simulink model "DSPB_MB_SS"  (Simulink 8.1)
settings: Solver=VariableStepDiscrete  StartTime=0.0  StopTime=DSPB_MB_SS_param.endTime  RelTol=1e-3
PreLoadFcn:
  | % Run the setup script when the model is opened
  | setup_DSPB_MB_SS;
InitFcn:
  | % Run the setup script again just before the
  | % model is run, so that any updates made
  | % after opening are applied.
  | setup_DSPB_MB_SS;
undefined symbols (not defined in the file or in its folder): a, AdvDSPBDMemDisplay, dpoly, DSPB_MB_SS_param, dspba, evalAionMaskParam, primtype, UseDontCare, value, x, y
libraries: DSPBAPrim x298, DspbAdvFftLibrary x34, DSPBABase x5, simulink x3, DSPBAModelBus x3, DSPBAVectorUtil x3, DSPBAControl x2
(part 1 of 4)
Description:
  | DSP Builder Advanced Template for Template Design implementing Primitive Subsystems
settings Model: Creator=mjervis  LastModifiedBy=AliReza
settings DataIOCC: SignalLoggingSaveFormat=Dataset
settings DebuggingCC: InheritedTsInSrcMsg=none  IntegerOverflowMsg=none  FcnCallInpInsideContextMsg=EnableAllAsError  FrameProcessingCompatibilityMsg=error
settings GRTTargetCC: CodeReplacementLibrary=None  CPPClassGenCompliant=on

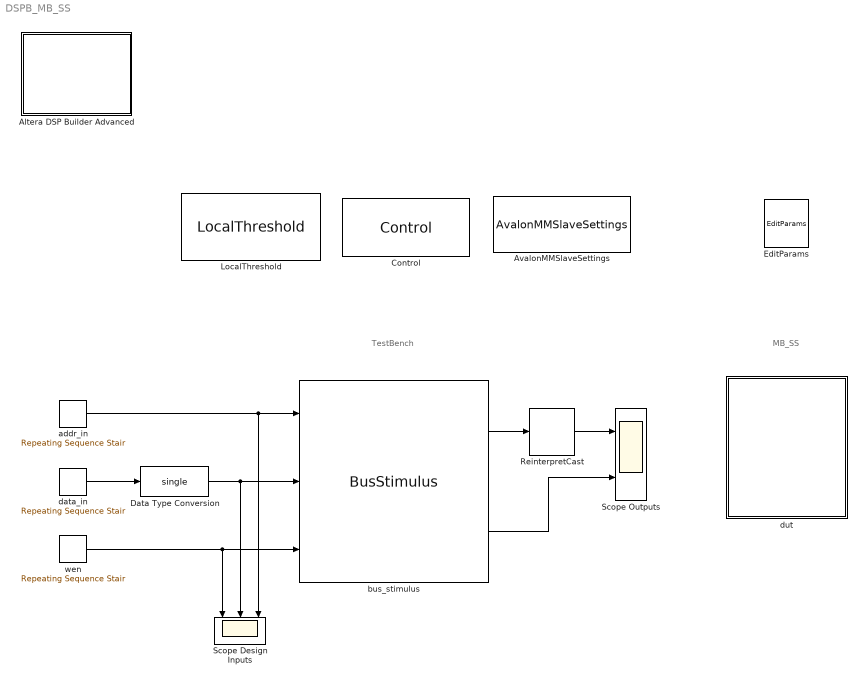
== system DSPB_MB_SS ==
  note: TestBench
  note: MB_SS
  Altera DSP Builder Advanced : Subsystem  mask(DSP Builder Advanced Blockset Ignored Block){}
      settings: OpenFcn=web('http://www.altera.com', '-new');
      mask Display: image(imread('intellogo.tif'));
  AvalonMMSlaveSettings : DSPBABase/AvalonMMSlaveSettings
  "Control " : DSPBABase/Control  generate=on  language=VHDL  destination=./rtl  make_full_path=off  path_is_relative=on  autotestbench=on  signaldepth=2  coveragetestbench=off  logs=off  spacewidth=2  spacenum=1  addrwidth=10  datawidth=16  dataendian=Big Endian  hierarchicalnames=on  ramThresholdBits=-1  distRamThresholdBits=-1  mlabThresholdBits=-1  hardMultiplierThresholdLuts=-1  version=20090407  errorOnChanMismatch=1  errorOnGPIOMismatch=0  importModelsimResults=0  cycleAccurate=off  reinterpretCastMult=off  paramFile=DSPB_MB_SS_params.xml
  Data Type Conversion : DataTypeConversion  OutDataTypeStr=single
  EditParams : DSPBABase/EditParams  version=20090407
  LocalThreshold : DSPBABase/LocalThreshold  margin=0  delayRegOrRAMThresholdBits=-1  MediumDualMemThresholdBits=-1  LargeDualMemThresholdBits=0  hardMultiplierThresholdLuts=0  complexMultKaratsuba=off  version=0
  ReinterpretCast : DSPBAPrim/ReinterpretCast  primtype=reinterpret  nInputs=1  nOutputs=1  omode=single  otype=sfix(16)  scale=2^-15  rndmethod=Unbiased  factor=1  satmethod=Symmetric  shift_vec=[0 1 2 -1]  value=0  inPortNames=[' '; ' ';]  outPortNames=[' ']  dspbaimage=dspba_prim.jpg  text=fprintf('Reinterp\nCast', value);  style=Optimised  visibilities=8  floatPrecision=float32_m23  version=20120601
  Scope Outputs : Scope  NumInputPorts=2
  Scope Design Inputs : Scope  NumInputPorts=3
  addr_in : simulink/Sources/Repeating Sequence Stair  OutValues=DSPB_MB_SS_IO.bus_addr_in  tsamp=1  OutMin=[]  OutMax=[]  OutDataTypeStr=Inherit: Inherit via back propagation  OutDataType=fixdt(0,3)  ConRadixGroup=Best Precision: Vector-wise  OutScaling=[]
  bus_stimulus : DSPBAModelBus/BusStimulus  SampleTime=-1  version=20140122  hasreaden=off
  data_in : simulink/Sources/Repeating Sequence Stair  OutValues=DSPB_MB_SS_IO.bus_data_in  tsamp=1  OutMin=[]  OutMax=[]  OutDataTypeStr=double  OutputDataTypeScalingMode=double  OutDataType=fixdt(0,3)  ConRadixGroup=Best Precision: Vector-wise  OutScaling=[]
  dut : Subsystem
  wen : simulink/Sources/Repeating Sequence Stair  OutValues=DSPB_MB_SS_IO.bus_wen  tsamp=1  OutMin=[]  OutMax=[]  OutDataTypeStr=fixdt('boolean')  OutputDataTypeScalingMode=Specify via dialog  OutDataType=fixdt('boolean')  ConRadixGroup=Best Precision: Vector-wise  OutScaling=[]
  wires:
  bus_stimulus/2 -> Scope Outputs/2
  addr_in/1 -> Scope Design Inputs/3, bus_stimulus/1
  wen/1 -> Scope Design Inputs/1, bus_stimulus/3
  data_in/1 -> Data Type Conversion/1
  Data Type Conversion/1 -> Scope Design Inputs/2, bus_stimulus/2
  bus_stimulus/1 -> ReinterpretCast/1
  ReinterpretCast/1 -> Scope Outputs/1

== system DSPB_MB_SS/Altera DSP Builder Advanced ==

== system DSPB_MB_SS/dut ==
  Device : DSPBABase/Device  family=Arria 10  stratix4device=Stratix IV E  hardcopy4device=HardCopy IV E  stratix5device=Stratix V GX  device=AUTO  speed=1  stratixSpeed=-5  stratix2Speed=-3  stratix3Speed=-2  stratix4gxSpeed=-2  stratix4gtSpeed=-1  cyclone2Speed=-6  cyclone3Speed=-7  arria2Speed=-4  cyclone4eSpeed=-8  stratix5Speed=-3  arria5Speed=-4  arriaSpeed=-6  cyclone3lsSpeed=-7  cyclone5Speed=-6  arria2gzSpeed=-3  nightFurySpeed=-2  ecp2Speed=-7  hardcopycompat=off  version=20140217  max10flashmode=off  max10nomeminit=off
  Enhacement_Algorithm_MB_SS : Subsystem
  Feature_Extraction : Subsystem
  Input_Interface : Subsystem
  Output_Interface : Subsystem
  wires:
  Feature_Extraction/1(Noisy_Signal_Power_Spectrum_Valid) -> Enhacement_Algorithm_MB_SS/1(Signal_Power_Spectrum_valid)
  Feature_Extraction/2(Noisy_Signal_Power_Spectrum) -> Enhacement_Algorithm_MB_SS/2(Signal_Power_Spectrum)
  Feature_Extraction/3(Noise_Power_Spectrum_Valid) -> Enhacement_Algorithm_MB_SS/3(Noise_Power_Spectrum_Valid)
  Feature_Extraction/5(Noisy_Signal_Phase_Valid) -> Enhacement_Algorithm_MB_SS/5(Signal_Phase_Valid)
  Feature_Extraction/6(Noisy_Signal_Phase) -> Enhacement_Algorithm_MB_SS/6(Signal_Phase)
  Enhacement_Algorithm_MB_SS/1(Enhanced_Signal_Valid) -> Output_Interface/1(Enhanced_Signal_Valid)
  Enhacement_Algorithm_MB_SS/2(Enhanced_Signal) -> Output_Interface/2(Enhanced_Signal)
  Input_Interface/1(Noisy_Signal_Valid) -> Feature_Extraction/1(Input_Signal_Valid)
  Feature_Extraction/4(Noise_Power_Spectrum) -> Enhacement_Algorithm_MB_SS/4(Noise_Power_Spectrum)
  Input_Interface/2(Noisy_Signal) -> Feature_Extraction/2(Input_Signal)

== system DSPB_MB_SS/dut/Enhacement_Algorithm_MB_SS ==
  Signal_Power_Spectrum_valid : Inport
  Signal_Power_Spectrum : Inport  Port=2
  Noise_Power_Spectrum_Valid : Inport  Port=3
  Noise_Power_Spectrum : Inport  Port=4
  Signal_Phase_Valid : Inport  Port=5
  Signal_Phase : Inport  Port=6
  MultiBand_Spectral_Subtraction : Subsystem
  Time_Domain_Reconstruction : Subsystem
  Enhanced_Signal_Valid : Outport
  Enhanced_Signal : Outport  Port=2
  wires:
  Time_Domain_Reconstruction/1(Time_Domain_Output_Valid) -> Enhanced_Signal_Valid/1
  Time_Domain_Reconstruction/2(Time_Domain_Output) -> Enhanced_Signal/1
  MultiBand_Spectral_Subtraction/1(Enhanced_Magnitude_Spectrum) -> Time_Domain_Reconstruction/1(Enhanced_Magnitude_Spectrum)
  MultiBand_Spectral_Subtraction/2(Enhanced_Magnitude_Spectrum_Valid) -> Time_Domain_Reconstruction/2(Enhanced_Magnitude_Spectrum_Valid)
  Noise_Power_Spectrum/1 -> MultiBand_Spectral_Subtraction/4(Noise_Power)
  Noise_Power_Spectrum_Valid/1 -> MultiBand_Spectral_Subtraction/3(Noise_Power_Valid)
  Signal_Power_Spectrum/1 -> MultiBand_Spectral_Subtraction/2(Signal_Power)
  Signal_Power_Spectrum_valid/1 -> MultiBand_Spectral_Subtraction/1(Signal_Power_Valid)
  Signal_Phase_Valid/1 -> Time_Domain_Reconstruction/3(Phase_Valid)
  Signal_Phase/1 -> Time_Domain_Reconstruction/4(Phase)

== system DSPB_MB_SS/dut/Feature_Extraction ==
  Input_Signal_Valid : Inport
  Input_Signal : Inport  Port=2
  A_Posteriori_SNR : Subsystem
  FFT : Subsystem
  FFT_Adapter : Subsystem
  Noisy_Signal_Power_Spectrum_Valid : Outport
  Noisy_Signal_Power_Spectrum : Outport  Port=2
  Noise_Power_Spectrum_Valid : Outport  Port=3
  Noise_Power_Spectrum : Outport  Port=4
  Noisy_Signal_Phase_Valid : Outport  Port=5
  Noisy_Signal_Phase : Outport  Port=6
  wires:
  FFT/1(_Valid) -> FFT_Adapter/1(FFT_In_Valid)
  FFT/2(Output) -> FFT_Adapter/2(FFT_In)
  A_Posteriori_SNR/1(Noise_Power_Spectrum_Valid) -> Noise_Power_Spectrum_Valid/1
  FFT_Adapter/1(Magnitude_Spectrum_Valid) -> A_Posteriori_SNR/1(Magnitude_Spectrum_Valid)
  FFT_Adapter/2(Magnitude_Spectrum) -> A_Posteriori_SNR/2(Magnitude_Spectrum)
  FFT_Adapter/5(Phase_Valid) -> Noisy_Signal_Phase_Valid/1
  FFT_Adapter/6(Phase) -> Noisy_Signal_Phase/1
  Input_Signal_Valid/1 -> FFT/1(Valid)
  Input_Signal/1 -> FFT/2(Input)
  FFT_Adapter/4(Power_Spectrum) -> Noisy_Signal_Power_Spectrum/1
  FFT_Adapter/3(Power_Spectrum_Valid) -> Noisy_Signal_Power_Spectrum_Valid/1
  A_Posteriori_SNR/2(Noise_Power_Spectrum) -> Noise_Power_Spectrum/1

== system DSPB_MB_SS/dut/Input_Interface ==
  And : DSPBAPrim/And  primtype=and  nInputs=3  nOutputs=1  omode=Inherit via internal rule  otype=sfix(16)  scale=2^-15  rndmethod=Unbiased  factor=1  satmethod=Symmetric  shift_vec=[0 1 2 -1]  value=0  inPortNames=[' '; ' '; ' '; ' '; ' '; ' '; ' '; ' '; ' '; ' '; ' '; ' '; ' '; ' '; ' '; ' '; ]  outPortNames=[' ']  dspbaimage=dspba_prim.jpg  text=fprintf('&');  style=Optimised  visibilities=8+2  version=20090407
  Const1 : DSPBAPrim/Const  primtype=const  nInputs=0  nOutputs=1  omode=Specify via dialog  otype=ufix(DSPB_MB_SS_param.FS+1)  scale=2^-0  rndmethod=Unbiased  factor=1  satmethod=Symmetric  shift_vec=[0 1 2 -1]  value=0  inPortNames=['+'; '+';]  outPortNames=[' ']  dspbaimage=dspba_prim.jpg  text=fprintf('%s', num2str(value));  style=Optimised  visibilities=8 + 1024  floatPrecision=float32_m23  version=20120820
  Const2 : DSPBAPrim/Const  primtype=const  nInputs=0  nOutputs=1  omode=single  otype=ufix(DSPB_MB_SS_param.FS+1)  scale=2^-0  rndmethod=Unbiased  factor=1  satmethod=Symmetric  shift_vec=[0 1 2 -1]  value=0  inPortNames=['+'; '+';]  outPortNames=[' ']  dspbaimage=dspba_prim.jpg  text=fprintf('%s', num2str(value));  style=Optimised  visibilities=8 + 1024  floatPrecision=float32_m23  version=20120820
  Const3 : DSPBAPrim/Const  primtype=const  nInputs=0  nOutputs=1  omode=single  otype=sfix(16)  scale=2^-15  rndmethod=Unbiased  factor=1  satmethod=Symmetric  shift_vec=[0 1 2 -1]  value=1  inPortNames=['+'; '+';]  outPortNames=[' ']  dspbaimage=dspba_prim.jpg  text=fprintf('%s', num2str(value));  style=Optimised  visibilities=8 + 1024  floatPrecision=float32_m23  version=20120820
  EdgeDetect : DspbAdvFftLibrary/Common/EdgeDetect
  GPOut : DSPBAPrim/GPOut  primtype=gpout  nInputs=evalAionMaskParam(gcb,'value',1)  nOutputs=evalAionMaskParam(gcb,'value',1)  omode=Inherit via internal rule  otype=sfix(16)  scale=2^-15  rndmethod=Unbiased  factor=1  satmethod=Symmetric  shift_vec=[0 1 2 -1]  value=2  inPortNames=[' ' ' ' ' ' ' ' ' ' ' ' ' ' ' ' ' ' ' ' ' ' ' ' ' ' ' ' ' ' ' ' ' ' ' ' ' ' ' ' ' ' ' ' ' ' ' ' ' ' ' ' ' ' ' ' ' ' ' ' ' ' ' ' ' ' ' ' ' ']'  outPortNames=[' ' ' ' ' ' ' ' ' ' ' ' ' ' ' ' ' ' ' ' ' ' ' ' ' ' ' ' ' ' ' ' ' ' ' ' ' ' ' ' ' ' ' ' ' ' ' ' ' ' ' ' ' ' ' ' ' ' ' ' ' ' ' ' ' ' ' ' ' ']'  dspbaimage=dspba_prim.jpg  text=fprintf('GPOut');  style=Optimised  visibilities=1024  latencyCorrection=0  version=20090407
  PulseMultiplier : DspbAdvFftLibrary/Common/PulseMultiplier  N=DSPB_MB_SS_param.FS
  SampleDelay : DSPBAPrim/SampleDelay  primtype=sampdelay  nInputs=1  nOutputs=1  omode=Inherit via internal rule  otype=sfix(16)  scale=2^-15  rndmethod=Unbiased  factor=1  satmethod=Symmetric  shift_vec=[0 1 2 -1]  value=3  inPortNames=[' '; ' ';]  outPortNames=[' ']  dspbaimage=dspba_prim.jpg  text=dpoly(1, eye(1,value+1), 'z')  style=Optimised  visibilities=8 + 1024 + 2^17 + 2^18  flexible=off  slackgroup=0  augmented=0  version=20090407  advOptions=[]
  SampleDelay1 : DSPBAPrim/SampleDelay  primtype=sampdelay  nInputs=1  nOutputs=1  omode=Inherit via internal rule  otype=sfix(16)  scale=2^-15  rndmethod=Unbiased  factor=1  satmethod=Symmetric  shift_vec=[0 1 2 -1]  value=1  inPortNames=[' '; ' ';]  outPortNames=[' ']  dspbaimage=dspba_prim.jpg  text=dpoly(1, eye(1,value+1), 'z')  style=Optimised  visibilities=8 + 1024 + 2^17 + 2^18  flexible=off  slackgroup=0  augmented=0  version=20090407  advOptions=[]
  SynthesisInfo : DSPBAPrim/SynthesisInfo  primtype=synthinfo  nInputs=0  nOutputs=0  omode=Inherit via internal rule  otype=sfix(16)  scale=2^-15  rndmethod=Truncate  factor=1  satmethod=Symmetric  shift_vec=[0 1 2 -1]  value=99  inPortNames=[' '; ' ';]  outPortNames=[' ']  dspbaimage=dspba_prim_ctrl.jpg  text=fprintf('Style=%s', style);  style=Scheduled  visibilities=2^17+2^18+2^19+2^20  constraintInUse=off  constraintRelation=>  constraintLimit=2  bitAccurate=off  version=20150220
  addr_counter : Subsystem
  frame_ready : DSPBAPrim/CmpEQ  primtype=cmpeq  nInputs=2  nOutputs=1  omode=boolean  otype=sfix(16)  scale=2^-15  rndmethod=Unbiased  factor=1  satmethod=Symmetric  shift_vec=[0 1 2 -1]  value=0  inPortNames=[' '; ' ';]  outPortNames=[' ']  dspbaimage=dspba_prim.jpg  text=fprintf('==');  style=Optimised  visibilities=0  advOptions=[]  version=20130117
  frame_ready1 : DSPBAPrim/CmpEQ  primtype=cmpeq  nInputs=2  nOutputs=1  omode=boolean  otype=sfix(16)  scale=2^-15  rndmethod=Unbiased  factor=1  satmethod=Symmetric  shift_vec=[0 1 2 -1]  value=0  inPortNames=[' '; ' ';]  outPortNames=[' ']  dspbaimage=dspba_prim.jpg  text=fprintf('==');  style=Optimised  visibilities=0  advOptions=[]  version=20130117
  input_fifo : DSPBAModelBus/SharedMem  mem_addr=0  mem_rwmode=Read/Write  mem_data=zeros(1,2^(DSPB_MB_SS_param.FS)+1)  mem_init=on  mem_desc=input fifo  mem_mode=single  mem_type=sfix(16)  mem_scale=2^-8  SampleTime=-1  version=20090407
  Noisy_Signal_Valid : Outport
  Noisy_Signal : Outport  Port=2
  wires:
  Const3/1 -> frame_ready/2
  And/1 -> SampleDelay/1
  SampleDelay/1 -> SampleDelay1/1, input_fifo/3
  addr_counter/1(count) -> input_fifo/1, frame_ready1/1
  SampleDelay1/1 -> PulseMultiplier/1
  frame_ready/1 -> EdgeDetect/1, And/1
  frame_ready1/1 -> And/2
  Const1/1 -> frame_ready1/2
  PulseMultiplier/1 -> GPOut/1, addr_counter/1(en)
  GPOut/2 -> Noisy_Signal/1
  EdgeDetect/1 -> And/3
  input_fifo/1 -> GPOut/2, frame_ready/1
  GPOut/1 -> Noisy_Signal_Valid/1
  Const2/1 -> input_fifo/2

== system DSPB_MB_SS/dut/Output_Interface ==
  Enhanced_Signal_Valid : Inport
  Enhanced_Signal : Inport  Port=2
  And2 : DSPBAPrim/And  primtype=and  nInputs=2  nOutputs=1  omode=Inherit via internal rule  otype=sfix(16)  scale=2^-15  rndmethod=Unbiased  factor=1  satmethod=Symmetric  shift_vec=[0 1 2 -1]  value=0  inPortNames=[' '; ' '; ' '; ' '; ' '; ' '; ' '; ' '; ' '; ' '; ' '; ' '; ' '; ' '; ' '; ' '; ]  outPortNames=[' ']  dspbaimage=dspba_prim.jpg  text=fprintf('&');  style=Optimised  visibilities=8+2  version=20090407
  Const : DSPBAPrim/Const  primtype=const  nInputs=0  nOutputs=1  omode=single  otype=sfix(16)  scale=2^-15  rndmethod=Unbiased  factor=1  satmethod=Symmetric  shift_vec=[0 1 2 -1]  value=1  inPortNames=['+'; '+';]  outPortNames=[' ']  dspbaimage=dspba_prim.jpg  text=fprintf('%s', num2str(value));  style=Optimised  visibilities=8 + 1024  floatPrecision=float32_m23  version=20120820
  DEBUG_MONITR : Subsystem  Commented=on
  EdgeDetect1 : DspbAdvFftLibrary/Common/EdgeDetect
  GPIn : DSPBAPrim/GPIn  primtype=gpin  nInputs=evalAionMaskParam(gcb,'value',1)  nOutputs=evalAionMaskParam(gcb,'value',1)  omode=Inherit via internal rule  otype=sfix(16)  scale=2^-15  rndmethod=Unbiased  factor=1  satmethod=Symmetric  shift_vec=[0 1 2 -1]  value=2  inPortNames=[' ' ' ' ' ' ' ' ' ' ' ' ' ' ' ' ' ' ' ' ' ' ' ' ' ' ' ' ' ' ' ' ' ' ' ' ' ' ' ' ' ' ' ' ' ' ' ' ' ' ' ' ' ' ' ' ' ' ' ' ' ' ' ' ' ' ' ' ' ']'  outPortNames=[' ' ' ' ' ' ' ' ' ' ' ' ' ' ' ' ' ' ' ' ' ' ' ' ' ' ' ' ' ' ' ' ' ' ' ' ' ' ' ' ' ' ' ' ' ' ' ' ' ' ' ' ' ' ' ' ' ' ' ' ' ' ' ' ' ' ' ' ' ']'  dspbaimage=dspba_prim.jpg  text=fprintf('GPIn');  style=Optimised  visibilities=1024  latencyCorrection=0  scheduleOrigin=on  version=20090407
  Mux : DSPBAPrim/Mux  primtype=mux  nInputs=evalAionMaskParam(gcb,'value',1)+1  nOutputs=1  omode=Inherit via internal rule  otype=sfix(16)  scale=2^-15  rndmethod=Unbiased  factor=1  satmethod=Symmetric  shift_vec=[0 1 2 -1]  value=2  inPortNames=['s '; 'd0'; 'd1'; 'd2'; 'd3'; 'd4'; 'd5'; 'd6'; 'd7'; 'd8'; 'd9';]  outPortNames=[' ']  dspbaimage=dspba_prim.jpg  text=fprintf('%s', primtype);  style=Optimised  visibilities=1032  version=20131025
  Not1 : DSPBAPrim/Not  primtype=not  nInputs=1  nOutputs=1  omode=Inherit via internal rule  otype=sfix(16)  scale=2^-15  rndmethod=Unbiased  factor=1  satmethod=Symmetric  shift_vec=[0 1 2 -1]  value=0  inPortNames=[' '; ' ';]  outPortNames=[' ']  dspbaimage=dspba_prim.jpg  text=fprintf('~');  style=Optimised  visibilities=8  version=20090407
  Or : DSPBAPrim/Or  primtype=or  nInputs=2  nOutputs=1  omode=Inherit via internal rule  otype=sfix(16)  scale=2^-15  rndmethod=Unbiased  factor=1  satmethod=Symmetric  shift_vec=[0 1 2 -1]  value=0  inPortNames=[' '; ' '; ' '; ' '; ' '; ' '; ' '; ' '; ' '; ' '; ' '; ' '; ' '; ' '; ' '; ' '; ]  outPortNames=[' ']  dspbaimage=dspba_prim.jpg  text=fprintf('|');  style=Optimised  visibilities=8+2  version=20090407
  SynthesisInfo : DSPBAPrim/SynthesisInfo  primtype=synthinfo  nInputs=0  nOutputs=0  omode=Inherit via internal rule  otype=sfix(16)  scale=2^-15  rndmethod=Truncate  factor=1  satmethod=Symmetric  shift_vec=[0 1 2 -1]  value=99  inPortNames=[' '; ' ';]  outPortNames=[' ']  dspbaimage=dspba_prim_ctrl.jpg  text=fprintf('Style=%s', style);  style=Scheduled  visibilities=2^17+2^18+2^19+2^20  constraintInUse=off  constraintRelation=>  constraintLimit=2  bitAccurate=off  version=20150220
  Terminator1 : Terminator
  addr_counter1 : Subsystem
  output_fifo : DSPBAModelBus/SharedMem  mem_addr=2^(DSPB_MB_SS_param.FS)+1  mem_rwmode=Read/Write  mem_data=zeros(1,2^(DSPB_MB_SS_param.FS)+1)  mem_init=on  mem_desc=output fifo  mem_mode=single  mem_type=sfix(16)  mem_scale=2^-8  SampleTime=-1  version=20090407
  wires:
  Enhanced_Signal/1 -> GPIn/2
  Enhanced_Signal_Valid/1 -> GPIn/1
  And2/1 -> Or/1, Mux/1
  GPIn/1 -> Or/2, Not1/1, EdgeDetect1/1, addr_counter1/1(en)
  output_fifo/1 -> Terminator1/1
  EdgeDetect1/1 -> And2/1
  Const/1 -> Mux/3
  Or/1 -> DEBUG_MONITR/3(we), output_fifo/3
  Not1/1 -> And2/2
  Mux/1 -> DEBUG_MONITR/2(wd), output_fifo/2
  GPIn/2 -> Mux/2
  addr_counter1/1(count) -> output_fifo/1, DEBUG_MONITR/1(addr)

== system DSPB_MB_SS/dut/Enhacement_Algorithm_MB_SS/MultiBand_Spectral_Subtraction ==
  note: S. D. Kamath and P. C. Loizou, “A MULTI-BAND SPECTRAL SUBTRACTION METHOD FOR ENHANCING SPEECH CORRUPTED BY COLORED NOISE,” p. 4.
  Signal_Power_Valid : Inport
  Signal_Power : Inport  Port=2
  Noise_Power_Valid : Inport  Port=3
  Noise_Power : Inport  Port=4
  Alpha : Subsystem
  MB_SS_Core : Subsystem
  Enhanced_Magnitude_Spectrum : Outport
  Enhanced_Magnitude_Spectrum_Valid : Outport  Port=2
  wires:
  Signal_Power/1 -> MB_SS_Core/2(Signal_Power), Alpha/2(Signal_Power)
  Signal_Power_Valid/1 -> MB_SS_Core/1(Signal_Power_Valid), Alpha/1(Signal_Power_Valid)
  Noise_Power_Valid/1 -> MB_SS_Core/3(Noise_Power_Valid), Alpha/3(Noise_Power_Valid)
  Noise_Power/1 -> MB_SS_Core/4(Noise_Power), Alpha/4(Noise_Power)
  Alpha/1(Valid) -> MB_SS_Core/5(Alpha_Valid)
  MB_SS_Core/1(Enhanced_Magnitude_Valid) -> Enhanced_Magnitude_Spectrum_Valid/1
  MB_SS_Core/2(Enhanced_Magnitude) -> Enhanced_Magnitude_Spectrum/1
  Alpha/2(Alpha) -> MB_SS_Core/6(Alpha)

== system DSPB_MB_SS/dut/Enhacement_Algorithm_MB_SS/Time_Domain_Reconstruction ==
  Enhanced_Magnitude_Spectrum : Inport
  Enhanced_Magnitude_Spectrum_Valid : Inport  Port=2
  Phase_Valid : Inport  Port=3
  Phase : Inport  Port=4
  IFFT : Subsystem
  IFFT_Adapter : Subsystem
  Time_Domain_Output_Valid : Outport
  Time_Domain_Output : Outport  Port=2
  wires:
  IFFT/2(Time_Domain_Output) -> Time_Domain_Output/1
  Enhanced_Magnitude_Spectrum_Valid/1 -> IFFT_Adapter/2(Enhanced_Magnitude_Valid)
  IFFT/1(Time_Domain_Output_Valid) -> Time_Domain_Output_Valid/1
  IFFT_Adapter/1(Output_Valid) -> IFFT/1(Input_Valid)
  IFFT_Adapter/2(Output) -> IFFT/2(Input)
  Enhanced_Magnitude_Spectrum/1 -> IFFT_Adapter/3(Enhanced_Magnitude)
  Phase_Valid/1 -> IFFT_Adapter/1(Phase_Valid)
  Phase/1 -> IFFT_Adapter/4(Phase)

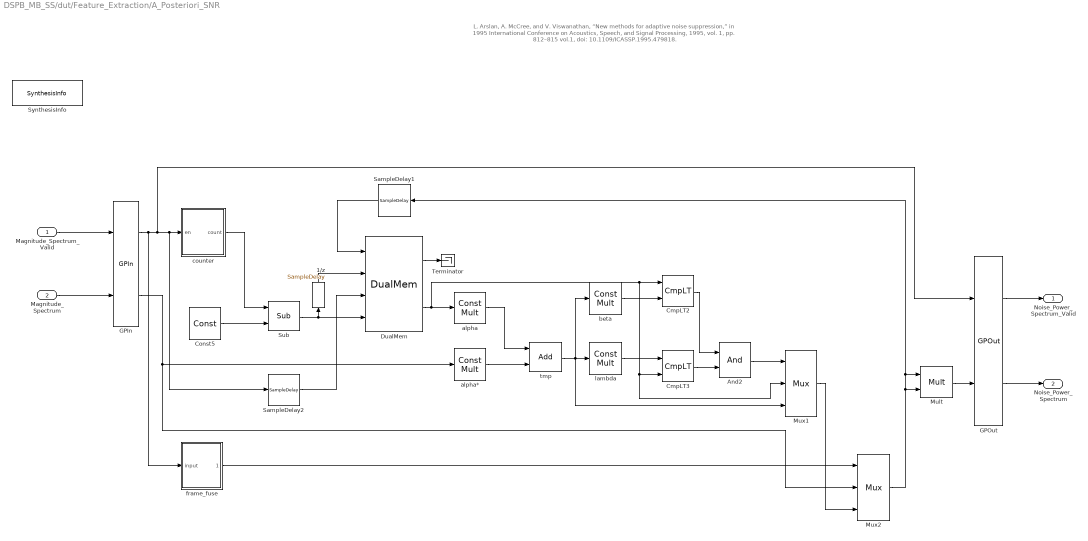
== system DSPB_MB_SS/dut/Feature_Extraction/A_Posteriori_SNR ==
  note: L. Arslan, A. McCree, and V. Viswanathan, “New methods for adaptive noise suppression,”
      |  in 1995 International Conference on Acoustics, Speech, and Signal Processing, 1995,
      | vol. 1, pp. 812–815 vol.1, doi: 10.1109/ICASSP.1995.479818.
  Magnitude_Spectrum_Valid : Inport
  Magnitude_Spectrum : Inport  Port=2
  1/z : DSPBAPrim/SampleDelay  primtype=sampdelay  nInputs=1  nOutputs=1  omode=Inherit via internal rule  otype=sfix(16)  scale=2^-15  rndmethod=Unbiased  factor=1  satmethod=Symmetric  shift_vec=[0 1 2 -1]  value=6  inPortNames=[' '; ' ';]  outPortNames=[' ']  dspbaimage=dspba_prim.jpg  text=dpoly(1, eye(1,value+1), 'z')  style=Optimised  visibilities=8 + 1024 + 2^17 + 2^18  flexible=off  slackgroup=0  augmented=0  version=20090407  advOptions=[]
  And2 : DSPBAPrim/And  primtype=and  nInputs=2  nOutputs=1  omode=Inherit via internal rule  otype=sfix(16)  scale=2^-15  rndmethod=Unbiased  factor=1  satmethod=Symmetric  shift_vec=[0 1 2 -1]  value=0  inPortNames=[' '; ' '; ' '; ' '; ' '; ' '; ' '; ' '; ' '; ' '; ' '; ' '; ' '; ' '; ' '; ' '; ]  outPortNames=[' ']  dspbaimage=dspba_prim.jpg  text=fprintf('&');  style=Optimised  visibilities=8+2  version=20090407
  CmpLT2 : DSPBAPrim/CmpLT  primtype=cmplt  nInputs=2  nOutputs=1  omode=boolean  otype=sfix(16)  scale=2^-15  rndmethod=Unbiased  factor=1  satmethod=Symmetric  shift_vec=[0 1 2 -1]  value=0  inPortNames=['a'; 'b';]  outPortNames=[' ']  dspbaimage=dspba_prim.jpg  text=fprintf('a<b');  style=Optimised  visibilities=0  advOptions=[]  version=20130117
  CmpLT3 : DSPBAPrim/CmpLT  primtype=cmplt  nInputs=2  nOutputs=1  omode=boolean  otype=sfix(16)  scale=2^-15  rndmethod=Unbiased  factor=1  satmethod=Symmetric  shift_vec=[0 1 2 -1]  value=0  inPortNames=['a'; 'b';]  outPortNames=[' ']  dspbaimage=dspba_prim.jpg  text=fprintf('a<b');  style=Optimised  visibilities=0  advOptions=[]  version=20130117
  Const5 : DSPBAPrim/Const  primtype=const  nInputs=0  nOutputs=1  omode=Specify via dialog  otype=ufix(DSPB_MB_SS_param.FS+1)  scale=2^-0  rndmethod=Unbiased  factor=1  satmethod=Symmetric  shift_vec=[0 1 2 -1]  value=1  inPortNames=['+'; '+';]  outPortNames=[' ']  dspbaimage=dspba_prim.jpg  text=fprintf('%s', num2str(value));  style=Optimised  visibilities=8 + 1024  floatPrecision=float32_m23  version=20120820
  DualMem : DSPBAPrim/DualMem  primtype=dualmem  nInputs=4  nOutputs=2  omode=single  otype=sfix(16)  scale=2^-15  rndmethod=Unbiased  factor=1  satmethod=Symmetric  shift_vec=[0 1 2 -1]  value=[zeros(2^DSPB_MB_SS_param.FS, 1)]  inPortNames=['d1'; 'a1'; 'w1'; 'a2']  outPortNames=['q1'; 'q2']  dspbaimage=dspba_prim.jpg  text=fprintf('dmem%s',AdvDSPBDMemDisplay(UseDontCare));  style=Optimised  visibilities=8 + 1024 + 2^17 + 2^18  UseDontCare=on  TwinWritePorts=off  version=20141001
  GPIn : DSPBAPrim/GPIn  primtype=gpin  nInputs=evalAionMaskParam(gcb,'value',1)  nOutputs=evalAionMaskParam(gcb,'value',1)  omode=Inherit via internal rule  otype=sfix(16)  scale=2^-15  rndmethod=Unbiased  factor=1  satmethod=Symmetric  shift_vec=[0 1 2 -1]  value=2  inPortNames=[' ' ' ' ' ' ' ' ' ' ' ' ' ' ' ' ' ' ' ' ' ' ' ' ' ' ' ' ' ' ' ' ' ' ' ' ' ' ' ' ' ' ' ' ' ' ' ' ' ' ' ' ' ' ' ' ' ' ' ' ' ' ' ' ' ' ' ' ' ']'  outPortNames=[' ' ' ' ' ' ' ' ' ' ' ' ' ' ' ' ' ' ' ' ' ' ' ' ' ' ' ' ' ' ' ' ' ' ' ' ' ' ' ' ' ' ' ' ' ' ' ' ' ' ' ' ' ' ' ' ' ' ' ' ' ' ' ' ' ' ' ' ' ']'  dspbaimage=dspba_prim.jpg  text=fprintf('GPIn');  style=Optimised  visibilities=1024  latencyCorrection=0  scheduleOrigin=on  version=20090407
  GPOut : DSPBAPrim/GPOut  primtype=gpout  nInputs=evalAionMaskParam(gcb,'value',1)  nOutputs=evalAionMaskParam(gcb,'value',1)  omode=Inherit via internal rule  otype=sfix(16)  scale=2^-15  rndmethod=Unbiased  factor=1  satmethod=Symmetric  shift_vec=[0 1 2 -1]  value=2  inPortNames=[' ' ' ' ' ' ' ' ' ' ' ' ' ' ' ' ' ' ' ' ' ' ' ' ' ' ' ' ' ' ' ' ' ' ' ' ' ' ' ' ' ' ' ' ' ' ' ' ' ' ' ' ' ' ' ' ' ' ' ' ' ' ' ' ' ' ' ' ' ']'  outPortNames=[' ' ' ' ' ' ' ' ' ' ' ' ' ' ' ' ' ' ' ' ' ' ' ' ' ' ' ' ' ' ' ' ' ' ' ' ' ' ' ' ' ' ' ' ' ' ' ' ' ' ' ' ' ' ' ' ' ' ' ' ' ' ' ' ' ' ' ' ' ']'  dspbaimage=dspba_prim.jpg  text=fprintf('GPOut');  style=Optimised  visibilities=1024  latencyCorrection=0  version=20090407
  Mult : DSPBAPrim/Mult  primtype=mult  nInputs=2  nOutputs=1  omode=Inherit via internal rule  otype=sfix(16)  scale=2^-15  rndmethod=Unbiased  factor=1  satmethod=Symmetric  shift_vec=[0 1 2 -1]  value=0  inPortNames=[' '; ' ';]  outPortNames=[' ']  dspbaimage=dspba_prim.jpg  text=fprintf('X');  style=Optimised  visibilities=8+2^18+2^19  floatPrecision=float32_m23  floatRounding=correct  advOptions=[]  version=20130115
  Mux1 : DSPBAPrim/Mux  primtype=mux  nInputs=evalAionMaskParam(gcb,'value',1)+1  nOutputs=1  omode=Inherit via internal rule  otype=sfix(16)  scale=2^-15  rndmethod=Unbiased  factor=1  satmethod=Symmetric  shift_vec=[0 1 2 -1]  value=2  inPortNames=['s '; 'd0'; 'd1'; 'd2'; 'd3'; 'd4'; 'd5'; 'd6'; 'd7'; 'd8'; 'd9';]  outPortNames=[' ']  dspbaimage=dspba_prim.jpg  text=fprintf('%s', primtype);  style=Optimised  visibilities=1032  version=20131025
  Mux2 : DSPBAPrim/Mux  primtype=mux  nInputs=evalAionMaskParam(gcb,'value',1)+1  nOutputs=1  omode=Inherit via internal rule  otype=sfix(16)  scale=2^-15  rndmethod=Unbiased  factor=1  satmethod=Symmetric  shift_vec=[0 1 2 -1]  value=2  inPortNames=['s '; 'd0'; 'd1'; 'd2'; 'd3'; 'd4'; 'd5'; 'd6'; 'd7'; 'd8'; 'd9';]  outPortNames=[' ']  dspbaimage=dspba_prim.jpg  text=fprintf('%s', primtype);  style=Optimised  visibilities=1032  version=20131025
  SampleDelay1 : DSPBAPrim/SampleDelay  primtype=sampdelay  nInputs=1  nOutputs=1  omode=Inherit via internal rule  otype=sfix(16)  scale=2^-15  rndmethod=Unbiased  factor=1  satmethod=Symmetric  shift_vec=[0 1 2 -1]  value=6  inPortNames=[' '; ' ';]  outPortNames=[' ']  dspbaimage=dspba_prim.jpg  text=dpoly(1, eye(1,value+1), 'z')  style=Optimised  visibilities=8 + 1024 + 2^17 + 2^18  flexible=off  slackgroup=0  augmented=0  version=20090407  advOptions=[]
  SampleDelay2 : DSPBAPrim/SampleDelay  primtype=sampdelay  nInputs=1  nOutputs=1  omode=Inherit via internal rule  otype=sfix(16)  scale=2^-15  rndmethod=Unbiased  factor=1  satmethod=Symmetric  shift_vec=[0 1 2 -1]  value=6  inPortNames=[' '; ' ';]  outPortNames=[' ']  dspbaimage=dspba_prim.jpg  text=dpoly(1, eye(1,value+1), 'z')  style=Optimised  visibilities=8 + 1024 + 2^17 + 2^18  flexible=off  slackgroup=0  augmented=0  version=20090407  advOptions=[]
  Sub : DSPBAPrim/Sub  primtype=sub  nInputs=2  nOutputs=1  omode=Specify via dialog  otype=ufix(DSPB_MB_SS_param.FS+1)  scale=2^-0  rndmethod=Unbiased  factor=1  satmethod=Symmetric  shift_vec=[0 1 2 -1]  value=0  inPortNames=['+'; '-';]  outPortNames=[' ']  dspbaimage=dspba_prim.jpg  text=fprintf('-');  style=Optimised  visibilities=8+2^17+2^18  floatRounding=correct  advOptions=[]  version=20130115
  SynthesisInfo : DSPBAPrim/SynthesisInfo  primtype=synthinfo  nInputs=0  nOutputs=0  omode=Inherit via internal rule  otype=sfix(16)  scale=2^-15  rndmethod=Truncate  factor=1  satmethod=Symmetric  shift_vec=[0 1 2 -1]  value=99  inPortNames=[' '; ' ';]  outPortNames=[' ']  dspbaimage=dspba_prim_ctrl.jpg  text=fprintf('Style=%s', style);  style=Scheduled  visibilities=2^17+2^18+2^19+2^20  constraintInUse=off  constraintRelation=<  constraintLimit=10000000  bitAccurate=on  version=20150220
  Terminator : Terminator
  alpha : DSPBAPrim/Const Mult  primtype=constmult  nInputs=1  nOutputs=1  omode=Inherit via internal rule  otype=sfix(16)  scale=2^-15  rndmethod=Unbiased  factor=1  satmethod=Symmetric  shift_vec=[0 1 2 -1]  value=0.9  inPortNames=[' '; ' ';]  outPortNames=[' ']  dspbaimage=dspba_prim.jpg  text=fprintf('cx');  style=Optimised  visibilities=8+2^10+2^17+2^18  floatRounding=correct  advOptions=[]  version=20140218
  alpha* : DSPBAPrim/Const Mult  primtype=constmult  nInputs=1  nOutputs=1  omode=Inherit via internal rule  otype=sfix(16)  scale=2^-15  rndmethod=Unbiased  factor=1  satmethod=Symmetric  shift_vec=[0 1 2 -1]  value=0.1  inPortNames=[' '; ' ';]  outPortNames=[' ']  dspbaimage=dspba_prim.jpg  text=fprintf('cx');  style=Optimised  visibilities=8+2^10+2^17+2^18  floatRounding=correct  advOptions=[]  version=20140218
  beta : DSPBAPrim/Const Mult  primtype=constmult  nInputs=1  nOutputs=1  omode=Inherit via internal rule  otype=sfix(16)  scale=2^-15  rndmethod=Unbiased  factor=1  satmethod=Symmetric  shift_vec=[0 1 2 -1]  value=1.2  inPortNames=[' '; ' ';]  outPortNames=[' ']  dspbaimage=dspba_prim.jpg  text=fprintf('cx');  style=Optimised  visibilities=8+2^10+2^17+2^18  floatRounding=correct  advOptions=[]  version=20140218
  counter : Subsystem
  frame_fuse : Subsystem
  lambda : DSPBAPrim/Const Mult  primtype=constmult  nInputs=1  nOutputs=1  omode=Inherit via internal rule  otype=sfix(16)  scale=2^-15  rndmethod=Unbiased  factor=1  satmethod=Symmetric  shift_vec=[0 1 2 -1]  value=0.85  inPortNames=[' '; ' ';]  outPortNames=[' ']  dspbaimage=dspba_prim.jpg  text=fprintf('cx');  style=Optimised  visibilities=8+2^10+2^17+2^18  floatRounding=correct  advOptions=[]  version=20140218
  tmp : DSPBAPrim/Add  primtype=add  nInputs=evalAionMaskParam(gcb,'value',1)  nOutputs=1  omode=Inherit via internal rule with word growth  otype=sfix(16)  scale=2^-15  rndmethod=Unbiased  factor=1  satmethod=Symmetric  shift_vec=[0 1 2 -1]  value=2  inPortNames=[' '; ' ';]  outPortNames=[' ']  dspbaimage=dspba_prim.jpg  text=fprintf('+');  style=Optimised  visibilities=1032+2^17+2^18+2^19  genFPC=off  floatRounding=correct  advOptions=[]  version=20130821
  Noise_Power_Spectrum_Valid : Outport
  Noise_Power_Spectrum : Outport  Port=2
  wires:
  Magnitude_Spectrum/1 -> GPIn/2
  Magnitude_Spectrum_Valid/1 -> GPIn/1
  GPIn/1 -> frame_fuse/1(input), GPOut/1, SampleDelay2/1, counter/1(en)
  counter/1(count) -> Sub/1
  Const5/1 -> Sub/2
  Sub/1 -> DualMem/4, 1/z/1
  GPIn/2 -> alpha*/1, Mux2/2
  DualMem/2 -> CmpLT2/1, Mux1/2, CmpLT3/2, alpha/1
  alpha*/1 -> tmp/2
  alpha/1 -> tmp/1
  tmp/1 -> beta/1, lambda/1, Mux1/3
  CmpLT2/1 -> And2/1
  CmpLT3/1 -> And2/2
  And2/1 -> Mux1/1
  beta/1 -> CmpLT2/2
  lambda/1 -> CmpLT3/1
  SampleDelay1/1 -> DualMem/1
  1/z/1 -> DualMem/2
  SampleDelay2/1 -> DualMem/3
  GPOut/1 -> Noise_Power_Spectrum_Valid/1
  GPOut/2 -> Noise_Power_Spectrum/1
  DualMem/1 -> Terminator/1
  frame_fuse/1(output) -> Mux2/1
  Mux1/1 -> Mux2/3
  Mux2/1 -> Mult/1, SampleDelay1/1, Mult/2
  Mult/1 -> GPOut/2

== system DSPB_MB_SS/dut/Feature_Extraction/FFT ==
  Valid : Inport
  Input : Inport  Port=2
  GPIn : DSPBAPrim/GPIn  primtype=gpin  nInputs=evalAionMaskParam(gcb,'value',1)  nOutputs=evalAionMaskParam(gcb,'value',1)  omode=Inherit via internal rule  otype=sfix(16)  scale=2^-15  rndmethod=Unbiased  factor=1  satmethod=Symmetric  shift_vec=[0 1 2 -1]  value=2  inPortNames=[' ' ' ' ' ' ' ' ' ' ' ' ' ' ' ' ' ' ' ' ' ' ' ' ' ' ' ' ' ' ' ' ' ' ' ' ' ' ' ' ' ' ' ' ' ' ' ' ' ' ' ' ' ' ' ' ' ' ' ' ' ' ' ' ' ' ' ' ' ']'  outPortNames=[' ' ' ' ' ' ' ' ' ' ' ' ' ' ' ' ' ' ' ' ' ' ' ' ' ' ' ' ' ' ' ' ' ' ' ' ' ' ' ' ' ' ' ' ' ' ' ' ' ' ' ' ' ' ' ' ' ' ' ' ' ' ' ' ' ' ' ' ' ']'  dspbaimage=dspba_prim.jpg  text=fprintf('GPIn');  style=Optimised  visibilities=1024  latencyCorrection=0  scheduleOrigin=on  version=20090407
  GPOut : DSPBAPrim/GPOut  primtype=gpout  nInputs=evalAionMaskParam(gcb,'value',1)  nOutputs=evalAionMaskParam(gcb,'value',1)  omode=Inherit via internal rule  otype=sfix(16)  scale=2^-15  rndmethod=Unbiased  factor=1  satmethod=Symmetric  shift_vec=[0 1 2 -1]  value=2  inPortNames=[' ' ' ' ' ' ' ' ' ' ' ' ' ' ' ' ' ' ' ' ' ' ' ' ' ' ' ' ' ' ' ' ' ' ' ' ' ' ' ' ' ' ' ' ' ' ' ' ' ' ' ' ' ' ' ' ' ' ' ' ' ' ' ' ' ' ' ' ' ']'  outPortNames=[' ' ' ' ' ' ' ' ' ' ' ' ' ' ' ' ' ' ' ' ' ' ' ' ' ' ' ' ' ' ' ' ' ' ' ' ' ' ' ' ' ' ' ' ' ' ' ' ' ' ' ' ' ' ' ' ' ' ' ' ' ' ' ' ' ' ' ' ' ']'  dspbaimage=dspba_prim.jpg  text=fprintf('GPOut');  style=Optimised  visibilities=1024  latencyCorrection=0  version=20090407
  SynthesisInfo : DSPBAPrim/SynthesisInfo  primtype=synthinfo  nInputs=0  nOutputs=0  omode=Inherit via internal rule  otype=sfix(16)  scale=2^-15  rndmethod=Truncate  factor=1  satmethod=Symmetric  shift_vec=[0 1 2 -1]  value=99  inPortNames=[' '; ' ';]  outPortNames=[' ']  dspbaimage=dspba_prim_ctrl.jpg  text=fprintf('Style=%s', style);  style=Scheduled  visibilities=32768  constraintInUse=off  constraintRelation=>  constraintLimit=2  bitAccurate=on  version=20150220
  Terminator : Terminator
  Terminator1 : Terminator
  bit_reversal : DspbAdvFftLibrary/Common/Transpose  perm=[fliplr(0:DSPB_MB_SS_param.FS-1)]
  float_fft : DspbAdvFftLibrary/Common/FFT_Light  IFFT=false  subchannels=1  br_in=true  N=DSPB_MB_SS_param.FS  in_type=dspba.namedVPFloat('single')  type_strings=dspba.fft.all_float(DSPB_MB_SS_param.FS,dspba.namedVPFloat('single'))  faithful=false  wirecount=1
  _Valid : Outport
  Output : Outport  Port=2
  wires:
  bit_reversal/3 -> Terminator/1
  bit_reversal/1 -> float_fft/1
  bit_reversal/2 -> float_fft/2
  float_fft/3 -> Terminator1/1
  GPIn/1 -> bit_reversal/1
  GPIn/2 -> bit_reversal/2
  Valid/1 -> GPIn/1
  Input/1 -> GPIn/2
  GPOut/1 -> _Valid/1
  GPOut/2 -> Output/1
  float_fft/1 -> GPOut/1
  float_fft/2 -> GPOut/2

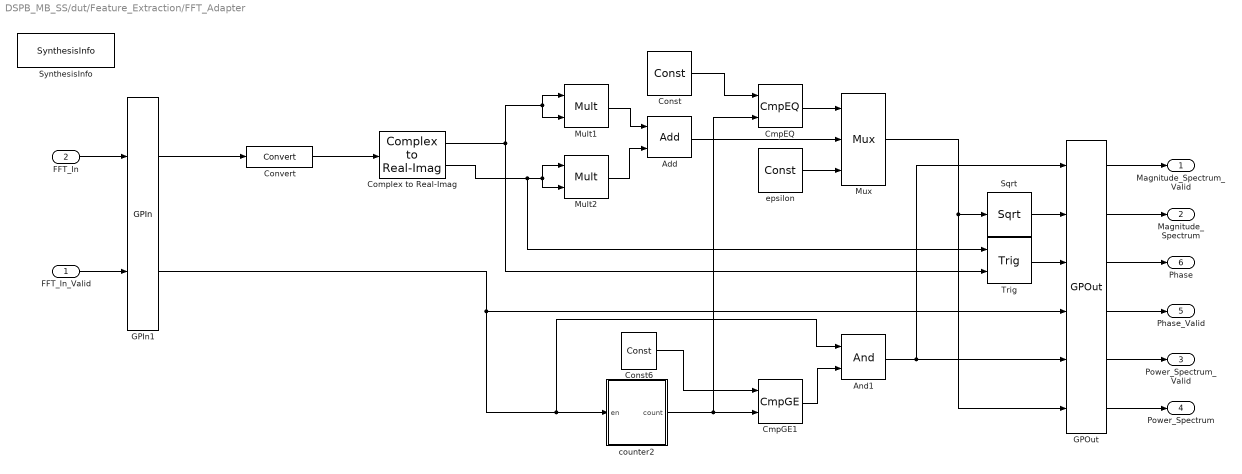
== system DSPB_MB_SS/dut/Feature_Extraction/FFT_Adapter ==
  FFT_In_Valid : Inport
  FFT_In : Inport  Port=2
  Add : DSPBAPrim/Add  primtype=add  nInputs=evalAionMaskParam(gcb,'value',1)  nOutputs=1  omode=Inherit via internal rule with word growth  otype=sfix(16)  scale=2^-15  rndmethod=Unbiased  factor=1  satmethod=Symmetric  shift_vec=[0 1 2 -1]  value=2  inPortNames=[' '; ' ';]  outPortNames=[' ']  dspbaimage=dspba_prim.jpg  text=fprintf('+');  style=Optimised  visibilities=1032+2^17+2^18+2^19  genFPC=off  floatRounding=correct  advOptions=[]  version=20130821
  And1 : DSPBAPrim/And  primtype=and  nInputs=2  nOutputs=1  omode=Inherit via internal rule  otype=sfix(16)  scale=2^-15  rndmethod=Unbiased  factor=1  satmethod=Symmetric  shift_vec=[0 1 2 -1]  value=0  inPortNames=[' '; ' '; ' '; ' '; ' '; ' '; ' '; ' '; ' '; ' '; ' '; ' '; ' '; ' '; ' '; ' '; ]  outPortNames=[' ']  dspbaimage=dspba_prim.jpg  text=fprintf('&');  style=Optimised  visibilities=8+2  version=20090407
  CmpEQ : DSPBAPrim/CmpEQ  primtype=cmpeq  nInputs=2  nOutputs=1  omode=boolean  otype=sfix(16)  scale=2^-15  rndmethod=Unbiased  factor=1  satmethod=Symmetric  shift_vec=[0 1 2 -1]  value=0  inPortNames=[' '; ' ';]  outPortNames=[' ']  dspbaimage=dspba_prim.jpg  text=fprintf('==');  style=Optimised  visibilities=0  advOptions=[]  version=20130117
  CmpGE1 : DSPBAPrim/CmpGE  primtype=cmpgte  nInputs=2  nOutputs=1  omode=boolean  otype=sfix(16)  scale=2^-15  rndmethod=Unbiased  factor=1  satmethod=Symmetric  shift_vec=[0 1 2 -1]  value=0  inPortNames=['a'; 'b';]  outPortNames=[' ']  dspbaimage=dspba_prim.jpg  text=fprintf('a>=b');  style=Optimised  visibilities=0  advOptions=[]  version=20130117
  Complex to Real-Imag : DSPBAVectorUtil/Complex to Real-Imag
  Const : DSPBAPrim/Const  primtype=const  nInputs=0  nOutputs=1  omode=Inherit via internal rule  otype=sfix(16)  scale=2^-15  rndmethod=Unbiased  factor=1  satmethod=Symmetric  shift_vec=[0 1 2 -1]  value=1  inPortNames=['+'; '+';]  outPortNames=[' ']  dspbaimage=dspba_prim.jpg  text=fprintf('%s', num2str(value));  style=Optimised  visibilities=8 + 1024  floatPrecision=float32_m23  version=20120820
  Const6 : DSPBAPrim/Const  primtype=const  nInputs=0  nOutputs=1  omode=Inherit via internal rule  otype=sfix(16)  scale=2^-15  rndmethod=Unbiased  factor=1  satmethod=Symmetric  shift_vec=[0 1 2 -1]  value=2^(DSPB_MB_SS_param.FS-1)  inPortNames=['+'; '+';]  outPortNames=[' ']  dspbaimage=dspba_prim.jpg  text=fprintf('%s', num2str(value));  style=Optimised  visibilities=8 + 1024  floatPrecision=float32_m23  version=20120820
  Convert : DSPBAPrim/Convert  primtype=convert  nInputs=1  nOutputs=1  omode=single  otype=sfix(16)  scale=2^-15  rndmethod=Biased  factor=1  satmethod=None  shift_vec=[0 1 2 -1]  value=round([0:255]/17)  inPortNames=[' '; ' ';]  outPortNames=[' '; 'c']  dspbaimage=dspba_prim.jpg  text=fprintf('convert');  style=Optimised  visibilities=8+64+256+2^17  clipdetect=off  floatPrecision=float32_m23  advOptions=[]  version=20130211
  GPIn1 : DSPBAPrim/GPIn  primtype=gpin  nInputs=evalAionMaskParam(gcb,'value',1)  nOutputs=evalAionMaskParam(gcb,'value',1)  omode=Inherit via internal rule  otype=sfix(16)  scale=2^-15  rndmethod=Unbiased  factor=1  satmethod=Symmetric  shift_vec=[0 1 2 -1]  value=2  inPortNames=[' ' ' ' ' ' ' ' ' ' ' ' ' ' ' ' ' ' ' ' ' ' ' ' ' ' ' ' ' ' ' ' ' ' ' ' ' ' ' ' ' ' ' ' ' ' ' ' ' ' ' ' ' ' ' ' ' ' ' ' ' ' ' ' ' ' ' ' ' ']'  outPortNames=[' ' ' ' ' ' ' ' ' ' ' ' ' ' ' ' ' ' ' ' ' ' ' ' ' ' ' ' ' ' ' ' ' ' ' ' ' ' ' ' ' ' ' ' ' ' ' ' ' ' ' ' ' ' ' ' ' ' ' ' ' ' ' ' ' ' ' ' ' ']'  dspbaimage=dspba_prim.jpg  text=fprintf('GPIn');  style=Optimised  visibilities=1024  latencyCorrection=0  scheduleOrigin=on  version=20090407
  GPOut : DSPBAPrim/GPOut  primtype=gpout  nInputs=evalAionMaskParam(gcb,'value',1)  nOutputs=evalAionMaskParam(gcb,'value',1)  omode=Inherit via internal rule  otype=sfix(16)  scale=2^-15  rndmethod=Unbiased  factor=1  satmethod=Symmetric  shift_vec=[0 1 2 -1]  value=6  inPortNames=[' ' ' ' ' ' ' ' ' ' ' ' ' ' ' ' ' ' ' ' ' ' ' ' ' ' ' ' ' ' ' ' ' ' ' ' ' ' ' ' ' ' ' ' ' ' ' ' ' ' ' ' ' ' ' ' ' ' ' ' ' ' ' ' ' ' ' ' ' ']'  outPortNames=[' ' ' ' ' ' ' ' ' ' ' ' ' ' ' ' ' ' ' ' ' ' ' ' ' ' ' ' ' ' ' ' ' ' ' ' ' ' ' ' ' ' ' ' ' ' ' ' ' ' ' ' ' ' ' ' ' ' ' ' ' ' ' ' ' ' ' ' ' ']'  dspbaimage=dspba_prim.jpg  text=fprintf('GPOut');  style=Optimised  visibilities=1024  latencyCorrection=0  version=20090407
  Mult1 : DSPBAPrim/Mult  primtype=mult  nInputs=2  nOutputs=1  omode=Inherit via internal rule  otype=sfix(16)  scale=2^-15  rndmethod=Unbiased  factor=1  satmethod=Symmetric  shift_vec=[0 1 2 -1]  value=0  inPortNames=[' '; ' ';]  outPortNames=[' ']  dspbaimage=dspba_prim.jpg  text=fprintf('X');  style=Optimised  visibilities=8+2^18+2^19  floatPrecision=float32_m23  floatRounding=correct  advOptions=[]  version=20130115
  Mult2 : DSPBAPrim/Mult  primtype=mult  nInputs=2  nOutputs=1  omode=Inherit via internal rule  otype=sfix(16)  scale=2^-15  rndmethod=Unbiased  factor=1  satmethod=Symmetric  shift_vec=[0 1 2 -1]  value=0  inPortNames=[' '; ' ';]  outPortNames=[' ']  dspbaimage=dspba_prim.jpg  text=fprintf('X');  style=Optimised  visibilities=8+2^18+2^19  floatPrecision=float32_m23  floatRounding=correct  advOptions=[]  version=20130115
  Mux : DSPBAPrim/Mux  primtype=mux  nInputs=evalAionMaskParam(gcb,'value',1)+1  nOutputs=1  omode=Inherit via internal rule  otype=sfix(16)  scale=2^-15  rndmethod=Unbiased  factor=1  satmethod=Symmetric  shift_vec=[0 1 2 -1]  value=2  inPortNames=['s '; 'd0'; 'd1'; 'd2'; 'd3'; 'd4'; 'd5'; 'd6'; 'd7'; 'd8'; 'd9';]  outPortNames=[' ']  dspbaimage=dspba_prim.jpg  text=fprintf('%s', primtype);  style=Optimised  visibilities=1032  version=20131025
  Sqrt : DSPBAPrim/Sqrt  primtype=sqrtfunc  nInputs=1  nOutputs=1  omode=Inherit via internal rule  otype=sfix(16)  scale=2^-15  rndmethod=Unbiased  factor=1  satmethod=Symmetric  shift_vec=[0 1 2 -1]  value=round([0:255]/17)  inPortNames=[' '; ' ';]  outPortNames=[' ']  dspbaimage=dspba_prim_float.jpg  text=fprintf('sqrt(x)');  style=Optimised  visibilities=2^17  functionExpr=sqrt(x)  floatRounding=correct  advOptions=[]  version=20120730
  SynthesisInfo : DSPBAPrim/SynthesisInfo  primtype=synthinfo  nInputs=0  nOutputs=0  omode=Inherit via internal rule  otype=sfix(16)  scale=2^-15  rndmethod=Truncate  factor=1  satmethod=Symmetric  shift_vec=[0 1 2 -1]  value=99  inPortNames=[' '; ' ';]  outPortNames=[' ']  dspbaimage=dspba_prim_ctrl.jpg  text=fprintf('Style=%s', style);  style=Scheduled  visibilities=2^17+2^18+2^19+2^20  constraintInUse=off  constraintRelation=>  constraintLimit=2  bitAccurate=on  version=20150220
  Trig : DSPBAPrim/Trig  primtype=trigfunc  nInputs=1  nOutputs=1  omode=Inherit via internal rule  otype=sfix(16)  scale=2^-15  rndmethod=Unbiased  factor=1  satmethod=Symmetric  shift_vec=[0 1 2 -1]  value=round([0:255]/17)  inPortNames=[' '; ' ';]  outPortNames=[' ']  dspbaimage=dspba_prim_float.jpg  text=fprintf('sin(a)');  style=Optimised  visibilities=2^17+2^18  functionExpr=atan2(y;x)  advOptions=[]  version=20140803
  counter2 : Subsystem
  epsilon : DSPBAPrim/Const  primtype=const  nInputs=0  nOutputs=1  omode=single  otype=sfix(16)  scale=2^-15  rndmethod=Unbiased  factor=1  satmethod=Symmetric  shift_vec=[0 1 2 -1]  value=2^-126  inPortNames=['+'; '+';]  outPortNames=[' ']  dspbaimage=dspba_prim.jpg  text=fprintf('%s', num2str(value));  style=Optimised  visibilities=8 + 1024  floatPrecision=float32_m23  version=20120820
  Magnitude_Spectrum_Valid : Outport
  Magnitude_Spectrum : Outport  Port=2
  Power_Spectrum_Valid : Outport  Port=3
  Power_Spectrum : Outport  Port=4
  Phase_Valid : Outport  Port=5
  Phase : Outport  Port=6
  wires:
  Mult1/1 -> Add/1
  Mult2/1 -> Add/2
  FFT_In_Valid/1 -> GPIn1/2
  FFT_In/1 -> GPIn1/1
  GPIn1/1 -> Convert/1
  Complex to Real-Imag/1 -> Mult1/2, Mult1/1, Trig/2
  Complex to Real-Imag/2 -> Trig/1, Mult2/2, Mult2/1
  Const6/1 -> CmpGE1/1
  counter2/1(count) -> CmpEQ/2, CmpGE1/2
  CmpGE1/1 -> And1/2
  And1/1 -> GPOut/5, GPOut/1
  Mux/1 -> GPOut/6, Sqrt/1
  Sqrt/1 -> GPOut/2
  Convert/1 -> Complex to Real-Imag/1
  Const/1 -> CmpEQ/1
  CmpEQ/1 -> Mux/1
  Add/1 -> Mux/2
  epsilon/1 -> Mux/3
  GPOut/1 -> Magnitude_Spectrum_Valid/1
  GPOut/2 -> Magnitude_Spectrum/1
  GPOut/3 -> Phase/1
  GPOut/4 -> Phase_Valid/1
  GPOut/5 -> Power_Spectrum_Valid/1
  GPOut/6 -> Power_Spectrum/1
  Trig/1 -> GPOut/3
  GPIn1/2 -> counter2/1(en), And1/1, GPOut/4

== system DSPB_MB_SS/dut/Input_Interface/addr_counter ==
  en : Inport
  CmpEQ : DSPBAPrim/CmpEQ  primtype=cmpeq  nInputs=2  nOutputs=1  omode=boolean  otype=sfix(16)  scale=2^-15  rndmethod=Unbiased  factor=1  satmethod=Symmetric  shift_vec=[0 1 2 -1]  value=0  inPortNames=[' '; ' ';]  outPortNames=[' ']  dspbaimage=dspba_prim.jpg  text=fprintf('==');  style=Optimised  visibilities=0  advOptions=[]  version=20130117
  Const1 : DSPBAPrim/Const  primtype=const  nInputs=0  nOutputs=1  omode=Specify via dialog  otype=ufix(DSPB_MB_SS_param.FS+1)  scale=2^-0  rndmethod=Unbiased  factor=1  satmethod=Symmetric  shift_vec=[0 1 2 -1]  value=2^(DSPB_MB_SS_param.FS) + 1  inPortNames=['+'; '+';]  outPortNames=[' ']  dspbaimage=dspba_prim.jpg  text=fprintf('%s', num2str(value));  style=Optimised  visibilities=8 + 1024  floatPrecision=float32_m23  version=20120820
  Const2 : DSPBAPrim/Const  primtype=const  nInputs=0  nOutputs=1  omode=Specify via dialog  otype=ufix(DSPB_MB_SS_param.FS + 1)  scale=2^-0  rndmethod=Unbiased  factor=1  satmethod=Symmetric  shift_vec=[0 1 2 -1]  value=2^(DSPB_MB_SS_param.FS)  inPortNames=['+'; '+';]  outPortNames=[' ']  dspbaimage=dspba_prim.jpg  text=fprintf('%s', num2str(value));  style=Optimised  visibilities=8 + 1024  floatPrecision=float32_m23  version=20120820
  Const3 : DSPBAPrim/Const  primtype=const  nInputs=0  nOutputs=1  omode=boolean  otype=ufix(10)  scale=2^-0  rndmethod=Unbiased  factor=1  satmethod=Symmetric  shift_vec=[0 1 2 -1]  value=1  inPortNames=['+'; '+';]  outPortNames=[' ']  dspbaimage=dspba_prim.jpg  text=fprintf('%s', num2str(value));  style=Optimised  visibilities=8 + 1024  floatPrecision=float32_m23  version=20120820
  Const4 : DSPBAPrim/Const  primtype=const  nInputs=0  nOutputs=1  omode=Inherit via internal rule  otype=ufix(10)  scale=2^-0  rndmethod=Unbiased  factor=1  satmethod=Symmetric  shift_vec=[0 1 2 -1]  value=0  inPortNames=['+'; '+';]  outPortNames=[' ']  dspbaimage=dspba_prim.jpg  text=fprintf('%s', num2str(value));  style=Optimised  visibilities=8 + 1024  floatPrecision=float32_m23  version=20120820
  LoadableCounter : DSPBAPrim/LoadableCounter  primtype=loadablecounter  nInputs=5  nOutputs=1  omode=Specify via dialog  otype=ufix(DSPB_MB_SS_param.FS+1)  scale=2^-0  rndmethod=Unbiased  factor=1  satmethod=Symmetric  shift_vec=[0 1 2 -1]  value=[0 2^(DSPB_MB_SS_param.FS) + 1 1]  inPortNames=['en';'ld';'i ';'s ';'m ']  outPortNames=[' ']  dspbaimage=dspba_prim.jpg  text=fprintf('loadable\ncounter\n[%d %d %d]', value(1), value(2), value(3));  style=Optimised  visibilities=8 + 1024  version=20090407
  SampleDelay : DSPBAPrim/SampleDelay  primtype=sampdelay  nInputs=1  nOutputs=1  omode=Inherit via internal rule  otype=sfix(16)  scale=2^-15  rndmethod=Unbiased  factor=1  satmethod=Symmetric  shift_vec=[0 1 2 -1]  value=1  inPortNames=[' '; ' ';]  outPortNames=[' ']  dspbaimage=dspba_prim.jpg  text=dpoly(1, eye(1,value+1), 'z')  style=Optimised  visibilities=8 + 1024 + 2^17 + 2^18  flexible=off  slackgroup=0  augmented=0  version=20090407  advOptions=[]
  count : Outport
  wires:
  Const2/1 -> CmpEQ/2
  CmpEQ/1 -> SampleDelay/1
  Const4/1 -> LoadableCounter/3
  Const1/1 -> LoadableCounter/5
  SampleDelay/1 -> LoadableCounter/2
  Const3/1 -> LoadableCounter/4
  en/1 -> LoadableCounter/1
  LoadableCounter/1 -> count/1, CmpEQ/1

== system DSPB_MB_SS/dut/Output_Interface/DEBUG_MONITR ==
  addr : Inport
  wd : Inport  Port=2
  we : Inport  Port=3
  And2 : DSPBAPrim/And  primtype=and  nInputs=3  nOutputs=1  omode=Inherit via internal rule  otype=sfix(16)  scale=2^-15  rndmethod=Unbiased  factor=1  satmethod=Symmetric  shift_vec=[0 1 2 -1]  value=0  inPortNames=[' '; ' '; ' '; ' '; ' '; ' '; ' '; ' '; ' '; ' '; ' '; ' '; ' '; ' '; ' '; ' '; ]  outPortNames=[' ']  dspbaimage=dspba_prim.jpg  text=fprintf('&');  style=Optimised  visibilities=8+2  version=20090407
  CmpLT : DSPBAPrim/CmpLT  primtype=cmplt  nInputs=2  nOutputs=1  omode=boolean  otype=sfix(16)  scale=2^-15  rndmethod=Unbiased  factor=1  satmethod=Symmetric  shift_vec=[0 1 2 -1]  value=0  inPortNames=['a'; 'b';]  outPortNames=[' ']  dspbaimage=dspba_prim.jpg  text=fprintf('a<b');  style=Optimised  visibilities=0  advOptions=[]  version=20130117
  CmpLT1 : DSPBAPrim/CmpLT  primtype=cmplt  nInputs=2  nOutputs=1  omode=boolean  otype=sfix(16)  scale=2^-15  rndmethod=Unbiased  factor=1  satmethod=Symmetric  shift_vec=[0 1 2 -1]  value=0  inPortNames=['a'; 'b';]  outPortNames=[' ']  dspbaimage=dspba_prim.jpg  text=fprintf('a<b');  style=Optimised  visibilities=0  advOptions=[]  version=20130117
  Const : DSPBAPrim/Const  primtype=const  nInputs=0  nOutputs=1  omode=single  otype=sfix(16)  scale=2^-15  rndmethod=Unbiased  factor=1  satmethod=Symmetric  shift_vec=[0 1 2 -1]  value=1234  inPortNames=['+'; '+';]  outPortNames=[' ']  dspbaimage=dspba_prim.jpg  text=fprintf('%s', num2str(value));  style=Optimised  visibilities=8 + 1024  floatPrecision=float32_m23  version=20120820
  Const1 : DSPBAPrim/Const  primtype=const  nInputs=0  nOutputs=1  omode=Inherit via internal rule  otype=sfix(16)  scale=2^-15  rndmethod=Unbiased  factor=1  satmethod=Symmetric  shift_vec=[0 1 2 -1]  value=401  inPortNames=['+'; '+';]  outPortNames=[' ']  dspbaimage=dspba_prim.jpg  text=fprintf('%s', num2str(value));  style=Optimised  visibilities=8 + 1024  floatPrecision=float32_m23  version=20120820
  Const2 : DSPBAPrim/Const  primtype=const  nInputs=0  nOutputs=1  omode=Inherit via internal rule  otype=sfix(16)  scale=2^-15  rndmethod=Unbiased  factor=1  satmethod=Symmetric  shift_vec=[0 1 2 -1]  value=1  inPortNames=['+'; '+';]  outPortNames=[' ']  dspbaimage=dspba_prim.jpg  text=fprintf('%s', num2str(value));  style=Optimised  visibilities=8 + 1024  floatPrecision=float32_m23  version=20120820
  Mux : DSPBAPrim/Mux  primtype=mux  nInputs=evalAionMaskParam(gcb,'value',1)+1  nOutputs=1  omode=Inherit via internal rule  otype=sfix(16)  scale=2^-15  rndmethod=Unbiased  factor=1  satmethod=Symmetric  shift_vec=[0 1 2 -1]  value=2  inPortNames=['s '; 'd0'; 'd1'; 'd2'; 'd3'; 'd4'; 'd5'; 'd6'; 'd7'; 'd8'; 'd9';]  outPortNames=[' ']  dspbaimage=dspba_prim.jpg  text=fprintf('%s', primtype);  style=Optimised  visibilities=1032  version=20131025
  Scope : Scope
      settings: TimeRange=5000  YMin=-0.2  YMax=0.225
  To Workspace : ToWorkspace  VariableName=out  SampleTime=-1
  latch_0L : DSPBAControl/latch_0L
  wires:
  addr/1 -> CmpLT1/2, CmpLT/1
  wd/1 -> latch_0L/2, Mux/3
  we/1 -> latch_0L/1, And2/2
  And2/1 -> Mux/1
  Mux/1 -> To Workspace/1
  Const/1 -> Mux/2
  latch_0L/1 -> Scope/1
  Const1/1 -> CmpLT/2
  CmpLT/1 -> And2/1
  Const2/1 -> CmpLT1/1
  CmpLT1/1 -> And2/3
